simulink model "DiagnosPipelineLogical"  (R2023b)
settings: Solver=VariableStepAuto  StartTime=0.0  StopTime=10.0  RelTol=1e-3
settings Model: Creator=user  LastModifiedBy=user

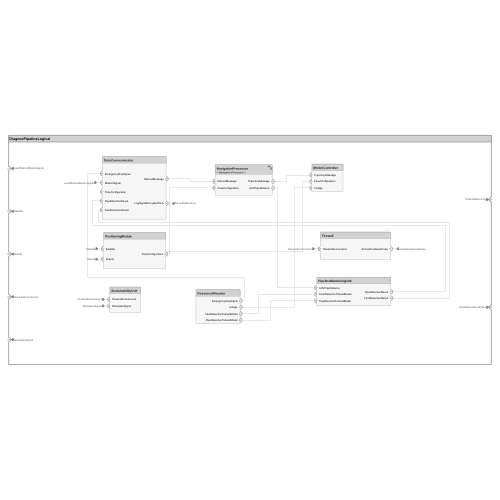
[thumbnail: Simulink's stored preview of the top-level diagram]
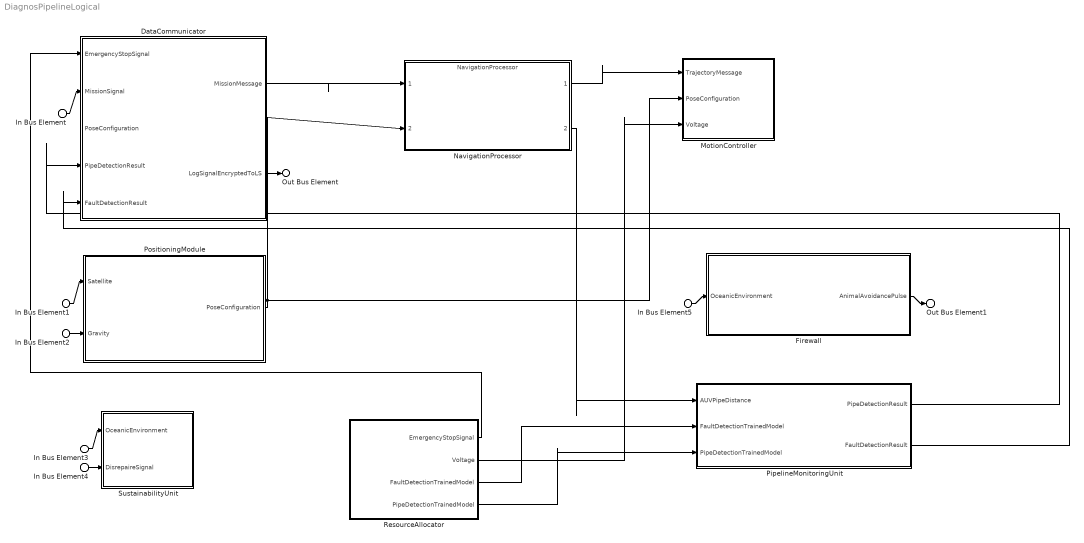
== system DiagnosPipelineLogical ==
  In Bus Element : Inport  PortName=LandStationMissionSignal
  In Bus Element1 : Inport  Port=2  PortName=Satellite
  In Bus Element2 : Inport  Port=3  PortName=Gravity
  In Bus Element3 : Inport  Port=4  PortName=OceanicEnvironment
  In Bus Element5 : Inport  Port=4  PortName=OceanicEnvironment
  In Bus Element4 : Inport  Port=5  PortName=DisrepaireSignal
  DataCommunicator : Subsystem
      settings: PortSchema="{\"entries\":[{\"content\":{\"headerSize\":26,\"margin\":15,\"minimumSpacing\":25,\"sides\":[{\"content\":{\"connectorIds\":[\"In1\",\"In2\",\"In3\",\"In4\",\"In5\"]},\"type\":\"ConnectorPlacement.EquallySpacedRectSide\",\"uuid\":\"f9fadc38-a5ed-4d2c-8740-325682f7523a\"},{\"content\":{\"connectorIds\":[\"Out1\",\"Out2\"],\"side\":\"RIGHT\"},\"type\":\"ConnectorPlacement.EquallySpacedRectSide\",\"uuid\":\"4cbd6435-b8f9-40e4-9703-696d88d9d9ae\"},{\"content\":{\"side\":\"TOP\"},\"type\":\"ConnectorPlacement.EquallySpacedRectSide\",\"uuid\":\"4cdd59a8-5a6d-4988-b682-29bfa74ce39c\"}]},\"type\":\"ConnectorPlacement.EquallySpacedConnector\",\"uuid\":\"f6db6523-916a-4ed8-a308-4b7cb9d0bc19\"}],\"packageUris\":[\"http://schema.mathworks.com/mf0/Connector/R2020b\"],\"version\":\"1.0\"}"
  Firewall : Subsystem
      settings: PortSchema="{\"entries\":[{\"content\":{\"headerSize\":26,\"margin\":15,\"minimumSpacing\":25,\"sides\":[{\"content\":{\"connectorIds\":[\"In1\"]},\"type\":\"ConnectorPlacement.EquallySpacedRectSide\",\"uuid\":\"f9fadc38-a5ed-4d2c-8740-325682f7523a\"},{\"content\":{\"connectorIds\":[\"Out1\"],\"side\":\"RIGHT\"},\"type\":\"ConnectorPlacement.EquallySpacedRectSide\",\"uuid\":\"4cbd6435-b8f9-40e4-9703-696d88d9d9ae\"},{\"content\":{\"side\":\"TOP\"},\"type\":\"ConnectorPlacement.EquallySpacedRectSide\",\"uuid\":\"4cdd59a8-5a6d-4988-b682-29bfa74ce39c\"}]},\"type\":\"ConnectorPlacement.EquallySpacedConnector\",\"uuid\":\"f6db6523-916a-4ed8-a308-4b7cb9d0bc19\"}],\"packageUris\":[\"http://schema.mathworks.com/mf0/Connector/R2020b\"],\"version\":\"1.0\"}"
  MotionController : Subsystem
      settings: PortSchema="{\"entries\":[{\"content\":{\"headerSize\":26,\"margin\":15,\"minimumSpacing\":25,\"sides\":[{\"content\":{\"connectorIds\":[\"In1\",\"In2\",\"In3\"]},\"type\":\"ConnectorPlacement.EquallySpacedRectSide\",\"uuid\":\"f9fadc38-a5ed-4d2c-8740-325682f7523a\"},{\"content\":{\"side\":\"RIGHT\"},\"type\":\"ConnectorPlacement.EquallySpacedRectSide\",\"uuid\":\"4cbd6435-b8f9-40e4-9703-696d88d9d9ae\"},{\"content\":{\"side\":\"TOP\"},\"type\":\"ConnectorPlacement.EquallySpacedRectSide\",\"uuid\":\"4cdd59a8-5a6d-4988-b682-29bfa74ce39c\"}]},\"type\":\"ConnectorPlacement.EquallySpacedConnector\",\"uuid\":\"f6db6523-916a-4ed8-a308-4b7cb9d0bc19\"}],\"packageUris\":[\"http://schema.mathworks.com/mf0/Connector/R2020b\"],\"version\":\"1.0\"}"
  NavigationProcessor : ModelReference  ModelNameDialog=NavigationProcessor  SimulationMode=Normal  ModelReferenceVersion=1.6
      settings: PortSchema="{\"entries\":[{\"content\":{\"headerSize\":38,\"margin\":15,\"minimumSpacing\":25,\"sides\":[{\"content\":{\"connectorIds\":[\"In1\",\"In2\"]},\"type\":\"ConnectorPlacement.EquallySpacedRectSide\",\"uuid\":\"f9fadc38-a5ed-4d2c-8740-325682f7523a\"},{\"content\":{\"connectorIds\":[\"Out1\",\"Out2\"],\"side\":\"RIGHT\"},\"type\":\"ConnectorPlacement.EquallySpacedRectSide\",\"uuid\":\"4cbd6435-b8f9-40e4-9703-696d88d9d9ae\"},{\"content\":{\"side\":\"TOP\"},\"type\":\"ConnectorPlacement.EquallySpacedRectSide\",\"uuid\":\"4cdd59a8-5a6d-4988-b682-29bfa74ce39c\"}]},\"type\":\"ConnectorPlacement.EquallySpacedConnector\",\"uuid\":\"f6db6523-916a-4ed8-a308-4b7cb9d0bc19\"}],\"packageUris\":[\"http://schema.mathworks.com/mf0/Connector/R2020b\"],\"version\":\"1.0\"}"
  PipelineMonitoringUnit : Subsystem
      settings: PortSchema="{\"entries\":[{\"content\":{\"headerSize\":26,\"margin\":15,\"minimumSpacing\":25,\"sides\":[{\"content\":{\"connectorIds\":[\"In1\",\"In2\",\"In3\"]},\"type\":\"ConnectorPlacement.EquallySpacedRectSide\",\"uuid\":\"f9fadc38-a5ed-4d2c-8740-325682f7523a\"},{\"content\":{\"connectorIds\":[\"Out1\",\"Out2\"],\"side\":\"RIGHT\"},\"type\":\"ConnectorPlacement.EquallySpacedRectSide\",\"uuid\":\"4cbd6435-b8f9-40e4-9703-696d88d9d9ae\"},{\"content\":{\"side\":\"TOP\"},\"type\":\"ConnectorPlacement.EquallySpacedRectSide\",\"uuid\":\"4cdd59a8-5a6d-4988-b682-29bfa74ce39c\"}]},\"type\":\"ConnectorPlacement.EquallySpacedConnector\",\"uuid\":\"f6db6523-916a-4ed8-a308-4b7cb9d0bc19\"}],\"packageUris\":[\"http://schema.mathworks.com/mf0/Connector/R2020b\"],\"version\":\"1.0\"}"
  PositioningModule : Subsystem
      settings: PortSchema="{\"entries\":[{\"content\":{\"headerSize\":26,\"margin\":15,\"minimumSpacing\":25,\"sides\":[{\"content\":{\"connectorIds\":[\"In1\",\"In2\"]},\"type\":\"ConnectorPlacement.EquallySpacedRectSide\",\"uuid\":\"f9fadc38-a5ed-4d2c-8740-325682f7523a\"},{\"content\":{\"connectorIds\":[\"Out1\"],\"side\":\"RIGHT\"},\"type\":\"ConnectorPlacement.EquallySpacedRectSide\",\"uuid\":\"4cbd6435-b8f9-40e4-9703-696d88d9d9ae\"},{\"content\":{\"side\":\"TOP\"},\"type\":\"ConnectorPlacement.EquallySpacedRectSide\",\"uuid\":\"4cdd59a8-5a6d-4988-b682-29bfa74ce39c\"}]},\"type\":\"ConnectorPlacement.EquallySpacedConnector\",\"uuid\":\"f6db6523-916a-4ed8-a308-4b7cb9d0bc19\"}],\"packageUris\":[\"http://schema.mathworks.com/mf0/Connector/R2020b\"],\"version\":\"1.0\"}"
  ResourceAllocator : Subsystem
      settings: PortSchema="{\"entries\":[{\"content\":{\"headerSize\":26,\"margin\":15,\"minimumSpacing\":25,\"sides\":[{\"content\":{},\"type\":\"ConnectorPlacement.EquallySpacedRectSide\",\"uuid\":\"f9fadc38-a5ed-4d2c-8740-325682f7523a\"},{\"content\":{\"connectorIds\":[\"Out3\",\"Out2\",\"Out1\",\"Out4\"],\"side\":\"RIGHT\"},\"type\":\"ConnectorPlacement.EquallySpacedRectSide\",\"uuid\":\"4cbd6435-b8f9-40e4-9703-696d88d9d9ae\"},{\"content\":{\"side\":\"TOP\"},\"type\":\"ConnectorPlacement.EquallySpacedRectSide\",\"uuid\":\"4cdd59a8-5a6d-4988-b682-29bfa74ce39c\"}]},\"type\":\"ConnectorPlacement.EquallySpacedConnector\",\"uuid\":\"f6db6523-916a-4ed8-a308-4b7cb9d0bc19\"}],\"packageUris\":[\"http://schema.mathworks.com/mf0/Connector/R2020b\"],\"version\":\"1.0\"}"
  SustainabilityUnit : Subsystem
      settings: PortSchema="{\"entries\":[{\"content\":{\"headerSize\":26,\"margin\":15,\"minimumSpacing\":25,\"sides\":[{\"content\":{\"connectorIds\":[\"In1\",\"In2\"]},\"type\":\"ConnectorPlacement.EquallySpacedRectSide\",\"uuid\":\"f9fadc38-a5ed-4d2c-8740-325682f7523a\"},{\"content\":{\"side\":\"RIGHT\"},\"type\":\"ConnectorPlacement.EquallySpacedRectSide\",\"uuid\":\"4cbd6435-b8f9-40e4-9703-696d88d9d9ae\"},{\"content\":{\"side\":\"TOP\"},\"type\":\"ConnectorPlacement.EquallySpacedRectSide\",\"uuid\":\"4cdd59a8-5a6d-4988-b682-29bfa74ce39c\"}]},\"type\":\"ConnectorPlacement.EquallySpacedConnector\",\"uuid\":\"f6db6523-916a-4ed8-a308-4b7cb9d0bc19\"}],\"packageUris\":[\"http://schema.mathworks.com/mf0/Connector/R2020b\"],\"version\":\"1.0\"}"
  Out Bus Element : Outport  PortName=ToLandStationLog
  Out Bus Element1 : Outport  Port=2  PortName=AnimalAvoidancePulse
  wires:
  In Bus Element/1 -> DataCommunicator/2(MissionSignal)
  DataCommunicator/2(LogSignalEncryptedToLS) -> Out Bus Element/1
  In Bus Element1/1 -> PositioningModule/1(Satellite)
  In Bus Element2/1 -> PositioningModule/2(Gravity)
  PositioningModule/1(PoseConfiguration) -> MotionController/2(PoseConfiguration), NavigationProcessor/2
  In Bus Element3/1 -> SustainabilityUnit/1(OceanicEnvironment)
  In Bus Element4/1 -> SustainabilityUnit/2(DisrepaireSignal)
  ResourceAllocator/2(Voltage) -> MotionController/3(Voltage)
  ResourceAllocator/3(EmergencyStopSignal) -> DataCommunicator/1(EmergencyStopSignal)
  ResourceAllocator/1(FaultDetectionTrainedModel) -> PipelineMonitoringUnit/2(FaultDetectionTrainedModel)
  ResourceAllocator/4(PipeDetectionTrainedModel) -> PipelineMonitoringUnit/3(PipeDetectionTrainedModel)
  PipelineMonitoringUnit/1(PipeDetectionResult) -> DataCommunicator/4(PipeDetectionResult)
  PipelineMonitoringUnit/2(FaultDetectionResult) -> DataCommunicator/5(FaultDetectionResult)
  In Bus Element5/1 -> Firewall/1(OceanicEnvironment)
  Firewall/1(AnimalAvoidancePulse) -> Out Bus Element1/1
  DataCommunicator/1(MissionMessage) -> NavigationProcessor/1
  NavigationProcessor/2 -> PipelineMonitoringUnit/1(AUVPipeDistance)
  NavigationProcessor/1 -> MotionController/1(TrajectoryMessage)

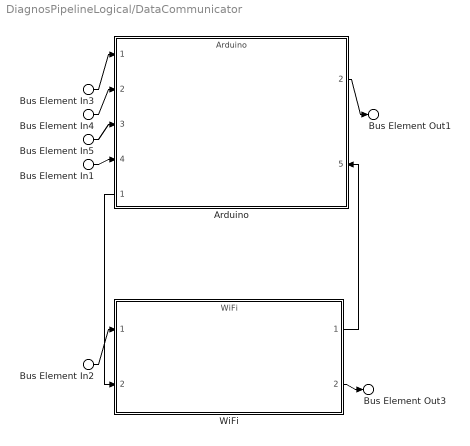
== system DiagnosPipelineLogical/DataCommunicator ==
  Bus Element In1 : Inport  PortName=EmergencyStopSignal
  Bus Element In2 : Inport  Port=2  PortName=MissionSignal
  Bus Element In3 : Inport  Port=3  PortName=PoseConfiguration
  Bus Element In4 : Inport  Port=4  PortName=PipeDetectionResult
  Bus Element In5 : Inport  Port=5  PortName=FaultDetectionResult
  Arduino : ModelReference  ModelNameDialog=Arduino  SimulationMode=Normal  ModelReferenceVersion=1.17
      settings: PortSchema="{\"entries\":[{\"content\":{\"headerSize\":38,\"margin\":15,\"minimumSpacing\":25,\"sides\":[{\"content\":{\"connectorIds\":[\"In1\",\"In2\",\"In3\",\"In4\",\"Out1\"]},\"type\":\"ConnectorPlacement.EquallySpacedRectSide\",\"uuid\":\"f9fadc38-a5ed-4d2c-8740-325682f7523a\"},{\"content\":{\"connectorIds\":[\"Out2\",\"In5\"],\"side\":\"RIGHT\"},\"type\":\"ConnectorPlacement.EquallySpacedRectSide\",\"uuid\":\"4cbd6435-b8f9-40e4-9703-696d88d9d9ae\"},{\"content\":{\"side\":\"TOP\"},\"type\":\"ConnectorPlacement.EquallySpacedRectSide\",\"uuid\":\"4cdd59a8-5a6d-4988-b682-29bfa74ce39c\"}]},\"type\":\"ConnectorPlacement.EquallySpacedConnector\",\"uuid\":\"f6db6523-916a-4ed8-a308-4b7cb9d0bc19\"}],\"packageUris\":[\"http://schema.mathworks.com/mf0/Connector/R2020b\"],\"version\":\"1.0\"}"
  WiFi : ModelReference  ModelNameDialog=WiFi  SimulationMode=Normal  ModelReferenceVersion=1.2
      settings: PortSchema="{\"entries\":[{\"content\":{\"headerSize\":38,\"margin\":15,\"minimumSpacing\":25,\"sides\":[{\"content\":{\"connectorIds\":[\"In1\",\"In2\"]},\"type\":\"ConnectorPlacement.EquallySpacedRectSide\",\"uuid\":\"f9fadc38-a5ed-4d2c-8740-325682f7523a\"},{\"content\":{\"connectorIds\":[\"Out1\",\"Out2\"],\"side\":\"RIGHT\"},\"type\":\"ConnectorPlacement.EquallySpacedRectSide\",\"uuid\":\"4cbd6435-b8f9-40e4-9703-696d88d9d9ae\"},{\"content\":{\"side\":\"TOP\"},\"type\":\"ConnectorPlacement.EquallySpacedRectSide\",\"uuid\":\"4cdd59a8-5a6d-4988-b682-29bfa74ce39c\"}]},\"type\":\"ConnectorPlacement.EquallySpacedConnector\",\"uuid\":\"f6db6523-916a-4ed8-a308-4b7cb9d0bc19\"}],\"packageUris\":[\"http://schema.mathworks.com/mf0/Connector/R2020b\"],\"version\":\"1.0\"}"
  Bus Element Out1 : Outport  PortName=MissionMessage
  Bus Element Out3 : Outport  Port=2  PortName=LogSignalEncryptedToLS
  wires:
  Bus Element In1/1 -> Arduino/4
  Bus Element In5/1 -> Arduino/3
  Bus Element In4/1 -> Arduino/2
  Bus Element In3/1 -> Arduino/1
  Arduino/2 -> Bus Element Out1/1
  Arduino/1 -> WiFi/2
  Bus Element In2/1 -> WiFi/1
  WiFi/2 -> Bus Element Out3/1
  WiFi/1 -> Arduino/5

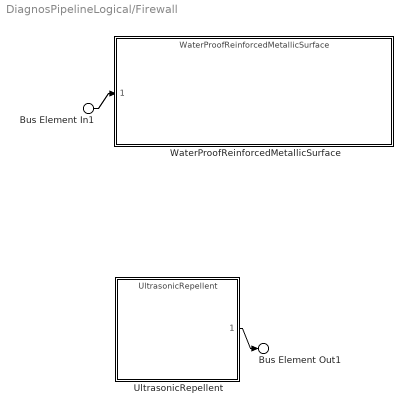
== system DiagnosPipelineLogical/Firewall ==
  Bus Element In1 : Inport  PortName=OceanicEnvironment
  UltrasonicRepellent : ModelReference  ModelNameDialog=UltrasonicRepellent  SimulationMode=Normal  ModelReferenceVersion=1.2
      settings: PortSchema="{\"entries\":[{\"content\":{\"headerSize\":38,\"margin\":15,\"minimumSpacing\":25,\"sides\":[{\"content\":{},\"type\":\"ConnectorPlacement.EquallySpacedRectSide\",\"uuid\":\"f9fadc38-a5ed-4d2c-8740-325682f7523a\"},{\"content\":{\"connectorIds\":[\"Out1\"],\"side\":\"RIGHT\"},\"type\":\"ConnectorPlacement.EquallySpacedRectSide\",\"uuid\":\"4cbd6435-b8f9-40e4-9703-696d88d9d9ae\"},{\"content\":{\"side\":\"TOP\"},\"type\":\"ConnectorPlacement.EquallySpacedRectSide\",\"uuid\":\"4cdd59a8-5a6d-4988-b682-29bfa74ce39c\"}]},\"type\":\"ConnectorPlacement.EquallySpacedConnector\",\"uuid\":\"f6db6523-916a-4ed8-a308-4b7cb9d0bc19\"}],\"packageUris\":[\"http://schema.mathworks.com/mf0/Connector/R2020b\"],\"version\":\"1.0\"}"
  WaterProofReinforcedMetallicSurface : ModelReference  ModelNameDialog=WaterProofReinforcedMetallicSurface  SimulationMode=Normal  ModelReferenceVersion=1.1
      settings: PortSchema="{\"entries\":[{\"content\":{\"headerSize\":38,\"margin\":15,\"minimumSpacing\":25,\"sides\":[{\"content\":{\"connectorIds\":[\"In1\"]},\"type\":\"ConnectorPlacement.EquallySpacedRectSide\",\"uuid\":\"f9fadc38-a5ed-4d2c-8740-325682f7523a\"},{\"content\":{\"side\":\"RIGHT\"},\"type\":\"ConnectorPlacement.EquallySpacedRectSide\",\"uuid\":\"4cbd6435-b8f9-40e4-9703-696d88d9d9ae\"},{\"content\":{\"side\":\"TOP\"},\"type\":\"ConnectorPlacement.EquallySpacedRectSide\",\"uuid\":\"4cdd59a8-5a6d-4988-b682-29bfa74ce39c\"}]},\"type\":\"ConnectorPlacement.EquallySpacedConnector\",\"uuid\":\"f6db6523-916a-4ed8-a308-4b7cb9d0bc19\"}],\"packageUris\":[\"http://schema.mathworks.com/mf0/Connector/R2020b\"],\"version\":\"1.0\"}"
  Bus Element Out1 : Outport  PortName=AnimalAvoidancePulse
  wires:
  Bus Element In1/1 -> WaterProofReinforcedMetallicSurface/1
  UltrasonicRepellent/1 -> Bus Element Out1/1

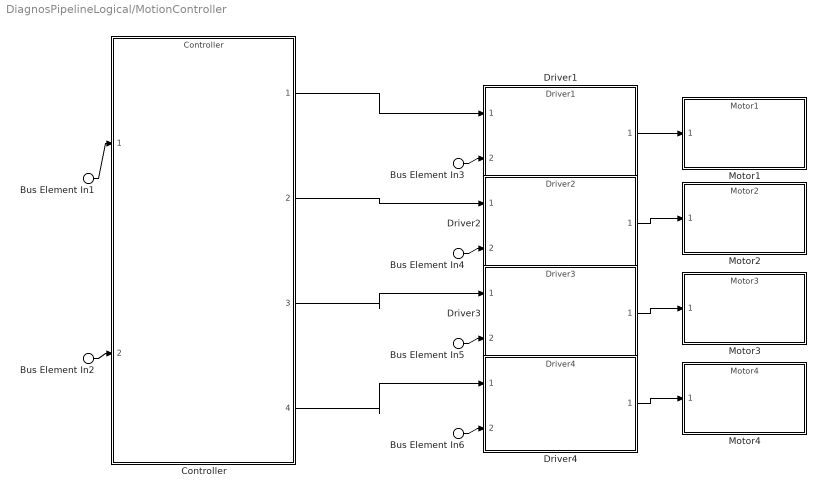
== system DiagnosPipelineLogical/MotionController ==
  Bus Element In1 : Inport  PortName=TrajectoryMessage
  Bus Element In2 : Inport  Port=2  PortName=PoseConfiguration
  Bus Element In{3..6} (4 alike) : Inport  Port=3  PortName=Voltage
  Controller : ModelReference  ModelNameDialog=Controller  SimulationMode=Normal  ModelReferenceVersion=1.2
      settings: PortSchema="{\"entries\":[{\"content\":{\"headerSize\":38,\"margin\":15,\"minimumSpacing\":25,\"sides\":[{\"content\":{\"connectorIds\":[\"In1\",\"In2\"]},\"type\":\"ConnectorPlacement.EquallySpacedRectSide\",\"uuid\":\"f9fadc38-a5ed-4d2c-8740-325682f7523a\"},{\"content\":{\"connectorIds\":[\"Out1\",\"Out2\",\"Out3\",\"Out4\"],\"side\":\"RIGHT\"},\"type\":\"ConnectorPlacement.EquallySpacedRectSide\",\"uuid\":\"4cbd6435-b8f9-40e4-9703-696d88d9d9ae\"},{\"content\":{\"side\":\"TOP\"},\"type\":\"ConnectorPlacement.EquallySpacedRectSide\",\"uuid\":\"4cdd59a8-5a6d-4988-b682-29bfa74ce39c\"}]},\"type\":\"ConnectorPlacement.EquallySpacedConnector\",\"uuid\":\"f6db6523-916a-4ed8-a308-4b7cb9d0bc19\"}],\"packageUris\":[\"http://schema.mathworks.com/mf0/Connector/R2020b\"],\"version\":\"1.0\"}"
  Driver1 : ModelReference  ModelNameDialog=Driver1  SimulationMode=Normal  ModelReferenceVersion=1.2
      settings: PortSchema="{\"entries\":[{\"content\":{\"headerSize\":38,\"margin\":15,\"minimumSpacing\":25,\"sides\":[{\"content\":{\"connectorIds\":[\"In1\",\"In2\"]},\"type\":\"ConnectorPlacement.EquallySpacedRectSide\",\"uuid\":\"f9fadc38-a5ed-4d2c-8740-325682f7523a\"},{\"content\":{\"connectorIds\":[\"Out1\"],\"side\":\"RIGHT\"},\"type\":\"ConnectorPlacement.EquallySpacedRectSide\",\"uuid\":\"4cbd6435-b8f9-40e4-9703-696d88d9d9ae\"},{\"content\":{\"side\":\"TOP\"},\"type\":\"ConnectorPlacement.EquallySpacedRectSide\",\"uuid\":\"4cdd59a8-5a6d-4988-b682-29bfa74ce39c\"}]},\"type\":\"ConnectorPlacement.EquallySpacedConnector\",\"uuid\":\"f6db6523-916a-4ed8-a308-4b7cb9d0bc19\"}],\"packageUris\":[\"http://schema.mathworks.com/mf0/Connector/R2020b\"],\"version\":\"1.0\"}"
  Driver2 : ModelReference  ModelNameDialog=Driver2  SimulationMode=Normal  ModelReferenceVersion=1.2
      settings: PortSchema="{\"entries\":[{\"content\":{\"headerSize\":38,\"margin\":15,\"minimumSpacing\":25,\"sides\":[{\"content\":{\"connectorIds\":[\"In1\",\"In2\"]},\"type\":\"ConnectorPlacement.EquallySpacedRectSide\",\"uuid\":\"f9fadc38-a5ed-4d2c-8740-325682f7523a\"},{\"content\":{\"connectorIds\":[\"Out1\"],\"side\":\"RIGHT\"},\"type\":\"ConnectorPlacement.EquallySpacedRectSide\",\"uuid\":\"4cbd6435-b8f9-40e4-9703-696d88d9d9ae\"},{\"content\":{\"side\":\"TOP\"},\"type\":\"ConnectorPlacement.EquallySpacedRectSide\",\"uuid\":\"4cdd59a8-5a6d-4988-b682-29bfa74ce39c\"}]},\"type\":\"ConnectorPlacement.EquallySpacedConnector\",\"uuid\":\"f6db6523-916a-4ed8-a308-4b7cb9d0bc19\"}],\"packageUris\":[\"http://schema.mathworks.com/mf0/Connector/R2020b\"],\"version\":\"1.0\"}"
  Driver3 : ModelReference  ModelNameDialog=Driver3  SimulationMode=Normal  ModelReferenceVersion=1.3
      settings: PortSchema="{\"entries\":[{\"content\":{\"headerSize\":38,\"margin\":15,\"minimumSpacing\":25,\"sides\":[{\"content\":{\"connectorIds\":[\"In1\",\"In2\"]},\"type\":\"ConnectorPlacement.EquallySpacedRectSide\",\"uuid\":\"f9fadc38-a5ed-4d2c-8740-325682f7523a\"},{\"content\":{\"connectorIds\":[\"Out1\"],\"side\":\"RIGHT\"},\"type\":\"ConnectorPlacement.EquallySpacedRectSide\",\"uuid\":\"4cbd6435-b8f9-40e4-9703-696d88d9d9ae\"},{\"content\":{\"side\":\"TOP\"},\"type\":\"ConnectorPlacement.EquallySpacedRectSide\",\"uuid\":\"4cdd59a8-5a6d-4988-b682-29bfa74ce39c\"}]},\"type\":\"ConnectorPlacement.EquallySpacedConnector\",\"uuid\":\"f6db6523-916a-4ed8-a308-4b7cb9d0bc19\"}],\"packageUris\":[\"http://schema.mathworks.com/mf0/Connector/R2020b\"],\"version\":\"1.0\"}"
  Driver4 : ModelReference  ModelNameDialog=Driver4  SimulationMode=Normal  ModelReferenceVersion=1.2
      settings: PortSchema="{\"entries\":[{\"content\":{\"headerSize\":38,\"margin\":15,\"minimumSpacing\":25,\"sides\":[{\"content\":{\"connectorIds\":[\"In1\",\"In2\"]},\"type\":\"ConnectorPlacement.EquallySpacedRectSide\",\"uuid\":\"f9fadc38-a5ed-4d2c-8740-325682f7523a\"},{\"content\":{\"connectorIds\":[\"Out1\"],\"side\":\"RIGHT\"},\"type\":\"ConnectorPlacement.EquallySpacedRectSide\",\"uuid\":\"4cbd6435-b8f9-40e4-9703-696d88d9d9ae\"},{\"content\":{\"side\":\"TOP\"},\"type\":\"ConnectorPlacement.EquallySpacedRectSide\",\"uuid\":\"4cdd59a8-5a6d-4988-b682-29bfa74ce39c\"}]},\"type\":\"ConnectorPlacement.EquallySpacedConnector\",\"uuid\":\"f6db6523-916a-4ed8-a308-4b7cb9d0bc19\"}],\"packageUris\":[\"http://schema.mathworks.com/mf0/Connector/R2020b\"],\"version\":\"1.0\"}"
  Motor1 : ModelReference  ModelNameDialog=Motor1  SimulationMode=Normal  ModelReferenceVersion=1.2
      settings: PortSchema="{\"entries\":[{\"content\":{\"headerSize\":38,\"margin\":15,\"minimumSpacing\":25,\"sides\":[{\"content\":{\"connectorIds\":[\"In1\"]},\"type\":\"ConnectorPlacement.EquallySpacedRectSide\",\"uuid\":\"f9fadc38-a5ed-4d2c-8740-325682f7523a\"},{\"content\":{\"side\":\"RIGHT\"},\"type\":\"ConnectorPlacement.EquallySpacedRectSide\",\"uuid\":\"4cbd6435-b8f9-40e4-9703-696d88d9d9ae\"},{\"content\":{\"side\":\"TOP\"},\"type\":\"ConnectorPlacement.EquallySpacedRectSide\",\"uuid\":\"4cdd59a8-5a6d-4988-b682-29bfa74ce39c\"}]},\"type\":\"ConnectorPlacement.EquallySpacedConnector\",\"uuid\":\"f6db6523-916a-4ed8-a308-4b7cb9d0bc19\"}],\"packageUris\":[\"http://schema.mathworks.com/mf0/Connector/R2020b\"],\"version\":\"1.0\"}"
  Motor2 : ModelReference  ModelNameDialog=Motor2  SimulationMode=Normal  ModelReferenceVersion=1.2
      settings: PortSchema="{\"entries\":[{\"content\":{\"headerSize\":38,\"margin\":15,\"minimumSpacing\":25,\"sides\":[{\"content\":{\"connectorIds\":[\"In1\"]},\"type\":\"ConnectorPlacement.EquallySpacedRectSide\",\"uuid\":\"f9fadc38-a5ed-4d2c-8740-325682f7523a\"},{\"content\":{\"side\":\"RIGHT\"},\"type\":\"ConnectorPlacement.EquallySpacedRectSide\",\"uuid\":\"4cbd6435-b8f9-40e4-9703-696d88d9d9ae\"},{\"content\":{\"side\":\"TOP\"},\"type\":\"ConnectorPlacement.EquallySpacedRectSide\",\"uuid\":\"4cdd59a8-5a6d-4988-b682-29bfa74ce39c\"}]},\"type\":\"ConnectorPlacement.EquallySpacedConnector\",\"uuid\":\"f6db6523-916a-4ed8-a308-4b7cb9d0bc19\"}],\"packageUris\":[\"http://schema.mathworks.com/mf0/Connector/R2020b\"],\"version\":\"1.0\"}"
  Motor3 : ModelReference  ModelNameDialog=Motor3  SimulationMode=Normal  ModelReferenceVersion=1.2
      settings: PortSchema="{\"entries\":[{\"content\":{\"headerSize\":38,\"margin\":15,\"minimumSpacing\":25,\"sides\":[{\"content\":{\"connectorIds\":[\"In1\"]},\"type\":\"ConnectorPlacement.EquallySpacedRectSide\",\"uuid\":\"f9fadc38-a5ed-4d2c-8740-325682f7523a\"},{\"content\":{\"side\":\"RIGHT\"},\"type\":\"ConnectorPlacement.EquallySpacedRectSide\",\"uuid\":\"4cbd6435-b8f9-40e4-9703-696d88d9d9ae\"},{\"content\":{\"side\":\"TOP\"},\"type\":\"ConnectorPlacement.EquallySpacedRectSide\",\"uuid\":\"4cdd59a8-5a6d-4988-b682-29bfa74ce39c\"}]},\"type\":\"ConnectorPlacement.EquallySpacedConnector\",\"uuid\":\"f6db6523-916a-4ed8-a308-4b7cb9d0bc19\"}],\"packageUris\":[\"http://schema.mathworks.com/mf0/Connector/R2020b\"],\"version\":\"1.0\"}"
  Motor4 : ModelReference  ModelNameDialog=Motor4  SimulationMode=Normal  ModelReferenceVersion=1.2
      settings: PortSchema="{\"entries\":[{\"content\":{\"headerSize\":38,\"margin\":15,\"minimumSpacing\":25,\"sides\":[{\"content\":{\"connectorIds\":[\"In1\"]},\"type\":\"ConnectorPlacement.EquallySpacedRectSide\",\"uuid\":\"f9fadc38-a5ed-4d2c-8740-325682f7523a\"},{\"content\":{\"side\":\"RIGHT\"},\"type\":\"ConnectorPlacement.EquallySpacedRectSide\",\"uuid\":\"4cbd6435-b8f9-40e4-9703-696d88d9d9ae\"},{\"content\":{\"side\":\"TOP\"},\"type\":\"ConnectorPlacement.EquallySpacedRectSide\",\"uuid\":\"4cdd59a8-5a6d-4988-b682-29bfa74ce39c\"}]},\"type\":\"ConnectorPlacement.EquallySpacedConnector\",\"uuid\":\"f6db6523-916a-4ed8-a308-4b7cb9d0bc19\"}],\"packageUris\":[\"http://schema.mathworks.com/mf0/Connector/R2020b\"],\"version\":\"1.0\"}"
  wires:
  Bus Element In2/1 -> Controller/2
  Bus Element In1/1 -> Controller/1
  Controller/1 -> Driver1/1
  Bus Element In3/1 -> Driver1/2
  Controller/2 -> Driver2/1
  Bus Element In4/1 -> Driver2/2
  Controller/3 -> Driver3/1
  Bus Element In5/1 -> Driver3/2
  Controller/4 -> Driver4/1
  Bus Element In6/1 -> Driver4/2
  Driver1/1 -> Motor1/1
  Driver2/1 -> Motor2/1
  Driver3/1 -> Motor3/1
  Driver4/1 -> Motor4/1

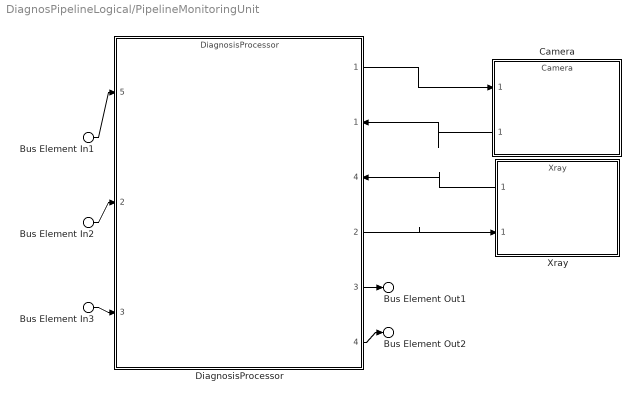
== system DiagnosPipelineLogical/PipelineMonitoringUnit ==
  Bus Element In1 : Inport  PortName=AUVPipeDistance
  Bus Element In2 : Inport  Port=2  PortName=FaultDetectionTrainedModel
  Bus Element In3 : Inport  Port=3  PortName=PipeDetectionTrainedModel
  Camera : ModelReference  ModelNameDialog=Camera  SimulationMode=Normal  ModelReferenceVersion=1.4
      settings: PortSchema="{\"entries\":[{\"content\":{\"headerSize\":38,\"margin\":15,\"minimumSpacing\":25,\"sides\":[{\"content\":{\"connectorIds\":[\"In1\",\"Out1\"]},\"type\":\"ConnectorPlacement.EquallySpacedRectSide\",\"uuid\":\"f9fadc38-a5ed-4d2c-8740-325682f7523a\"},{\"content\":{\"side\":\"RIGHT\"},\"type\":\"ConnectorPlacement.EquallySpacedRectSide\",\"uuid\":\"4cbd6435-b8f9-40e4-9703-696d88d9d9ae\"},{\"content\":{\"side\":\"TOP\"},\"type\":\"ConnectorPlacement.EquallySpacedRectSide\",\"uuid\":\"4cdd59a8-5a6d-4988-b682-29bfa74ce39c\"}]},\"type\":\"ConnectorPlacement.EquallySpacedConnector\",\"uuid\":\"f6db6523-916a-4ed8-a308-4b7cb9d0bc19\"}],\"packageUris\":[\"http://schema.mathworks.com/mf0/Connector/R2020b\"],\"version\":\"1.0\"}"
  DiagnosisProcessor : ModelReference  ModelNameDialog=DiagnosisProcessor  SimulationMode=Normal  ModelReferenceVersion=1.3
      settings: PortSchema="{\"entries\":[{\"content\":{\"headerSize\":38,\"margin\":15,\"minimumSpacing\":25,\"sides\":[{\"content\":{\"connectorIds\":[\"In5\",\"In2\",\"In3\"]},\"type\":\"ConnectorPlacement.EquallySpacedRectSide\",\"uuid\":\"f9fadc38-a5ed-4d2c-8740-325682f7523a\"},{\"content\":{\"connectorIds\":[\"Out1\",\"In1\",\"In4\",\"Out2\",\"Out3\",\"Out4\"],\"side\":\"RIGHT\"},\"type\":\"ConnectorPlacement.EquallySpacedRectSide\",\"uuid\":\"4cbd6435-b8f9-40e4-9703-696d88d9d9ae\"},{\"content\":{\"side\":\"TOP\"},\"type\":\"ConnectorPlacement.EquallySpacedRectSide\",\"uuid\":\"4cdd59a8-5a6d-4988-b682-29bfa74ce39c\"}]},\"type\":\"ConnectorPlacement.EquallySpacedConnector\",\"uuid\":\"f6db6523-916a-4ed8-a308-4b7cb9d0bc19\"}],\"packageUris\":[\"http://schema.mathworks.com/mf0/Connector/R2020b\"],\"version\":\"1.0\"}"
  Xray : ModelReference  ModelNameDialog=Xray  SimulationMode=Normal  ModelReferenceVersion=1.2
      settings: PortSchema="{\"entries\":[{\"content\":{\"headerSize\":38,\"margin\":15,\"minimumSpacing\":25,\"sides\":[{\"content\":{\"connectorIds\":[\"Out1\",\"In1\"]},\"type\":\"ConnectorPlacement.EquallySpacedRectSide\",\"uuid\":\"f9fadc38-a5ed-4d2c-8740-325682f7523a\"},{\"content\":{\"side\":\"RIGHT\"},\"type\":\"ConnectorPlacement.EquallySpacedRectSide\",\"uuid\":\"4cbd6435-b8f9-40e4-9703-696d88d9d9ae\"},{\"content\":{\"side\":\"TOP\"},\"type\":\"ConnectorPlacement.EquallySpacedRectSide\",\"uuid\":\"4cdd59a8-5a6d-4988-b682-29bfa74ce39c\"}]},\"type\":\"ConnectorPlacement.EquallySpacedConnector\",\"uuid\":\"f6db6523-916a-4ed8-a308-4b7cb9d0bc19\"}],\"packageUris\":[\"http://schema.mathworks.com/mf0/Connector/R2020b\"],\"version\":\"1.0\"}"
  Bus Element Out1 : Outport  PortName=PipeDetectionResult
  Bus Element Out2 : Outport  Port=2  PortName=FaultDetectionResult
  wires:
  Bus Element In1/1 -> DiagnosisProcessor/5
  Bus Element In2/1 -> DiagnosisProcessor/2
  Bus Element In3/1 -> DiagnosisProcessor/3
  DiagnosisProcessor/4 -> Bus Element Out2/1
  DiagnosisProcessor/3 -> Bus Element Out1/1
  DiagnosisProcessor/1 -> Camera/1
  Camera/1 -> DiagnosisProcessor/1
  DiagnosisProcessor/2 -> Xray/1
  Xray/1 -> DiagnosisProcessor/4

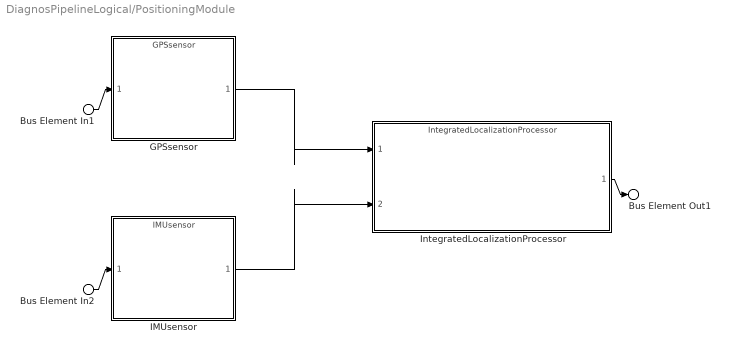
== system DiagnosPipelineLogical/PositioningModule ==
  Bus Element In1 : Inport  PortName=Satellite
  Bus Element In2 : Inport  Port=2  PortName=Gravity
  GPSsensor : ModelReference  ModelNameDialog=GPSsensor  SimulationMode=Normal  ModelReferenceVersion=1.3
      settings: PortSchema="{\"entries\":[{\"content\":{\"headerSize\":38,\"margin\":15,\"minimumSpacing\":25,\"sides\":[{\"content\":{\"connectorIds\":[\"In1\"]},\"type\":\"ConnectorPlacement.EquallySpacedRectSide\",\"uuid\":\"f9fadc38-a5ed-4d2c-8740-325682f7523a\"},{\"content\":{\"connectorIds\":[\"Out1\"],\"side\":\"RIGHT\"},\"type\":\"ConnectorPlacement.EquallySpacedRectSide\",\"uuid\":\"4cbd6435-b8f9-40e4-9703-696d88d9d9ae\"},{\"content\":{\"side\":\"TOP\"},\"type\":\"ConnectorPlacement.EquallySpacedRectSide\",\"uuid\":\"4cdd59a8-5a6d-4988-b682-29bfa74ce39c\"}]},\"type\":\"ConnectorPlacement.EquallySpacedConnector\",\"uuid\":\"f6db6523-916a-4ed8-a308-4b7cb9d0bc19\"}],\"packageUris\":[\"http://schema.mathworks.com/mf0/Connector/R2020b\"],\"version\":\"1.0\"}"
  IMUsensor : ModelReference  ModelNameDialog=IMUsensor  SimulationMode=Normal  ModelReferenceVersion=1.5
      settings: PortSchema="{\"entries\":[{\"content\":{\"headerSize\":38,\"margin\":15,\"minimumSpacing\":25,\"sides\":[{\"content\":{\"connectorIds\":[\"In1\"]},\"type\":\"ConnectorPlacement.EquallySpacedRectSide\",\"uuid\":\"f9fadc38-a5ed-4d2c-8740-325682f7523a\"},{\"content\":{\"connectorIds\":[\"Out1\"],\"side\":\"RIGHT\"},\"type\":\"ConnectorPlacement.EquallySpacedRectSide\",\"uuid\":\"4cbd6435-b8f9-40e4-9703-696d88d9d9ae\"},{\"content\":{\"side\":\"TOP\"},\"type\":\"ConnectorPlacement.EquallySpacedRectSide\",\"uuid\":\"4cdd59a8-5a6d-4988-b682-29bfa74ce39c\"}]},\"type\":\"ConnectorPlacement.EquallySpacedConnector\",\"uuid\":\"f6db6523-916a-4ed8-a308-4b7cb9d0bc19\"}],\"packageUris\":[\"http://schema.mathworks.com/mf0/Connector/R2020b\"],\"version\":\"1.0\"}"
  IntegratedLocalizationProcessor : ModelReference  ModelNameDialog=IntegratedLocalizationProcessor  SimulationMode=Normal  ModelReferenceVersion=1.25
      settings: PortSchema="{\"entries\":[{\"content\":{\"headerSize\":38,\"margin\":15,\"minimumSpacing\":25,\"sides\":[{\"content\":{\"connectorIds\":[\"In1\",\"In2\"]},\"type\":\"ConnectorPlacement.EquallySpacedRectSide\",\"uuid\":\"f9fadc38-a5ed-4d2c-8740-325682f7523a\"},{\"content\":{\"connectorIds\":[\"Out1\"],\"side\":\"RIGHT\"},\"type\":\"ConnectorPlacement.EquallySpacedRectSide\",\"uuid\":\"4cbd6435-b8f9-40e4-9703-696d88d9d9ae\"},{\"content\":{\"side\":\"TOP\"},\"type\":\"ConnectorPlacement.EquallySpacedRectSide\",\"uuid\":\"4cdd59a8-5a6d-4988-b682-29bfa74ce39c\"}]},\"type\":\"ConnectorPlacement.EquallySpacedConnector\",\"uuid\":\"f6db6523-916a-4ed8-a308-4b7cb9d0bc19\"}],\"packageUris\":[\"http://schema.mathworks.com/mf0/Connector/R2020b\"],\"version\":\"1.0\"}"
  Bus Element Out1 : Outport  PortName=PoseConfiguration
  wires:
  Bus Element In1/1 -> GPSsensor/1
  Bus Element In2/1 -> IMUsensor/1
  IMUsensor/1 -> IntegratedLocalizationProcessor/2
  GPSsensor/1 -> IntegratedLocalizationProcessor/1
  IntegratedLocalizationProcessor/1 -> Bus Element Out1/1

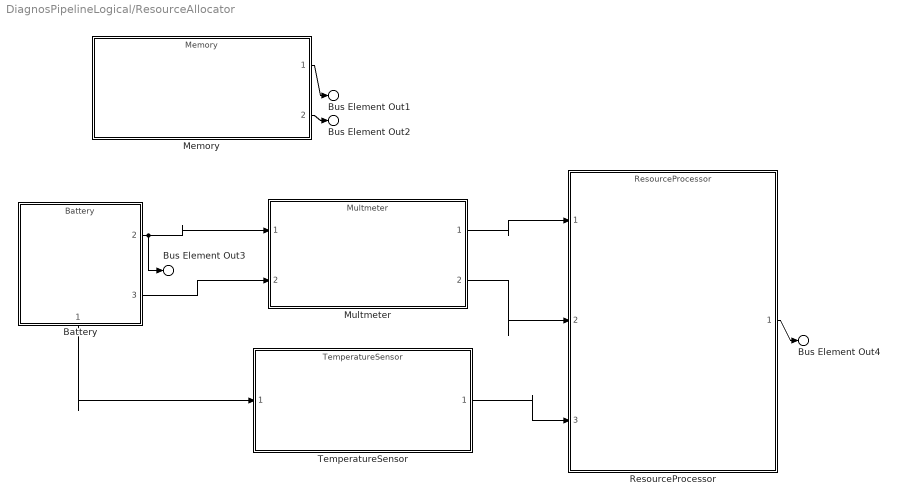
== system DiagnosPipelineLogical/ResourceAllocator ==
  Battery : ModelReference  ModelNameDialog=Battery  SimulationMode=Normal  ModelReferenceVersion=1.3
      settings: PortSchema="{\"entries\":[{\"content\":{\"headerSize\":38,\"margin\":15,\"minimumSpacing\":25,\"sides\":[{\"content\":{},\"type\":\"ConnectorPlacement.EquallySpacedRectSide\",\"uuid\":\"f9fadc38-a5ed-4d2c-8740-325682f7523a\"},{\"content\":{\"connectorIds\":[\"Out2\",\"Out3\"],\"side\":\"RIGHT\"},\"type\":\"ConnectorPlacement.EquallySpacedRectSide\",\"uuid\":\"4cbd6435-b8f9-40e4-9703-696d88d9d9ae\"},{\"content\":{\"side\":\"TOP\"},\"type\":\"ConnectorPlacement.EquallySpacedRectSide\",\"uuid\":\"4cdd59a8-5a6d-4988-b682-29bfa74ce39c\"},{\"content\":{\"connectorIds\":[\"Out1\"],\"side\":\"BOTTOM\"},\"type\":\"ConnectorPlacement.EquallySpacedRectSide\",\"uuid\":\"54b9e8e1-ed1a-443b-b89e-f595aeddcba4\"}]},\"type\":\"ConnectorPlacement.EquallySpacedConnector\",\"uuid\":\"f6db6523-916a-4ed8-a308-4b7cb9d0bc19\"}],\"packageUris\":[\"http://schema.mathworks.com/mf0/Connector/R2020b\"],\"version\":\"1.0\"}"
  Memory : ModelReference  ModelNameDialog=Memory  SimulationMode=Normal  ModelReferenceVersion=1.2
      settings: PortSchema="{\"entries\":[{\"content\":{\"headerSize\":38,\"margin\":15,\"minimumSpacing\":25,\"sides\":[{\"content\":{},\"type\":\"ConnectorPlacement.EquallySpacedRectSide\",\"uuid\":\"f9fadc38-a5ed-4d2c-8740-325682f7523a\"},{\"content\":{\"connectorIds\":[\"Out1\",\"Out2\"],\"side\":\"RIGHT\"},\"type\":\"ConnectorPlacement.EquallySpacedRectSide\",\"uuid\":\"4cbd6435-b8f9-40e4-9703-696d88d9d9ae\"},{\"content\":{\"side\":\"TOP\"},\"type\":\"ConnectorPlacement.EquallySpacedRectSide\",\"uuid\":\"4cdd59a8-5a6d-4988-b682-29bfa74ce39c\"}]},\"type\":\"ConnectorPlacement.EquallySpacedConnector\",\"uuid\":\"f6db6523-916a-4ed8-a308-4b7cb9d0bc19\"}],\"packageUris\":[\"http://schema.mathworks.com/mf0/Connector/R2020b\"],\"version\":\"1.0\"}"
  Multmeter : ModelReference  ModelNameDialog=Multmeter  SimulationMode=Normal  ModelReferenceVersion=1.2
      settings: PortSchema="{\"entries\":[{\"content\":{\"headerSize\":38,\"margin\":15,\"minimumSpacing\":25,\"sides\":[{\"content\":{\"connectorIds\":[\"In1\",\"In2\"]},\"type\":\"ConnectorPlacement.EquallySpacedRectSide\",\"uuid\":\"f9fadc38-a5ed-4d2c-8740-325682f7523a\"},{\"content\":{\"connectorIds\":[\"Out1\",\"Out2\"],\"side\":\"RIGHT\"},\"type\":\"ConnectorPlacement.EquallySpacedRectSide\",\"uuid\":\"4cbd6435-b8f9-40e4-9703-696d88d9d9ae\"},{\"content\":{\"side\":\"TOP\"},\"type\":\"ConnectorPlacement.EquallySpacedRectSide\",\"uuid\":\"4cdd59a8-5a6d-4988-b682-29bfa74ce39c\"}]},\"type\":\"ConnectorPlacement.EquallySpacedConnector\",\"uuid\":\"f6db6523-916a-4ed8-a308-4b7cb9d0bc19\"}],\"packageUris\":[\"http://schema.mathworks.com/mf0/Connector/R2020b\"],\"version\":\"1.0\"}"
  ResourceProcessor : ModelReference  ModelNameDialog=ResourceProcessor  SimulationMode=Normal  ModelReferenceVersion=1.2
      settings: PortSchema="{\"entries\":[{\"content\":{\"headerSize\":38,\"margin\":15,\"minimumSpacing\":25,\"sides\":[{\"content\":{\"connectorIds\":[\"In1\",\"In2\",\"In3\"]},\"type\":\"ConnectorPlacement.EquallySpacedRectSide\",\"uuid\":\"f9fadc38-a5ed-4d2c-8740-325682f7523a\"},{\"content\":{\"connectorIds\":[\"Out1\"],\"side\":\"RIGHT\"},\"type\":\"ConnectorPlacement.EquallySpacedRectSide\",\"uuid\":\"4cbd6435-b8f9-40e4-9703-696d88d9d9ae\"},{\"content\":{\"side\":\"TOP\"},\"type\":\"ConnectorPlacement.EquallySpacedRectSide\",\"uuid\":\"4cdd59a8-5a6d-4988-b682-29bfa74ce39c\"}]},\"type\":\"ConnectorPlacement.EquallySpacedConnector\",\"uuid\":\"f6db6523-916a-4ed8-a308-4b7cb9d0bc19\"}],\"packageUris\":[\"http://schema.mathworks.com/mf0/Connector/R2020b\"],\"version\":\"1.0\"}"
  TemperatureSensor : ModelReference  ModelNameDialog=TemperatureSensor  SimulationMode=Normal  ModelReferenceVersion=1.2
      settings: PortSchema="{\"entries\":[{\"content\":{\"headerSize\":38,\"margin\":15,\"minimumSpacing\":25,\"sides\":[{\"content\":{\"connectorIds\":[\"In1\"]},\"type\":\"ConnectorPlacement.EquallySpacedRectSide\",\"uuid\":\"f9fadc38-a5ed-4d2c-8740-325682f7523a\"},{\"content\":{\"connectorIds\":[\"Out1\"],\"side\":\"RIGHT\"},\"type\":\"ConnectorPlacement.EquallySpacedRectSide\",\"uuid\":\"4cbd6435-b8f9-40e4-9703-696d88d9d9ae\"},{\"content\":{\"side\":\"TOP\"},\"type\":\"ConnectorPlacement.EquallySpacedRectSide\",\"uuid\":\"4cdd59a8-5a6d-4988-b682-29bfa74ce39c\"}]},\"type\":\"ConnectorPlacement.EquallySpacedConnector\",\"uuid\":\"f6db6523-916a-4ed8-a308-4b7cb9d0bc19\"}],\"packageUris\":[\"http://schema.mathworks.com/mf0/Connector/R2020b\"],\"version\":\"1.0\"}"
  Bus Element Out2 : Outport  PortName=FaultDetectionTrainedModel
  Bus Element Out3 : Outport  Port=2  PortName=Voltage
  Bus Element Out4 : Outport  Port=3  PortName=EmergencyStopSignal
  Bus Element Out1 : Outport  Port=4  PortName=PipeDetectionTrainedModel
  wires:
  Memory/2 -> Bus Element Out2/1
  Memory/1 -> Bus Element Out1/1
  Battery/2 -> Bus Element Out3/1, Multmeter/1
  Battery/3 -> Multmeter/2
  Battery/1 -> TemperatureSensor/1
  Multmeter/2 -> ResourceProcessor/2
  TemperatureSensor/1 -> ResourceProcessor/3
  Multmeter/1 -> ResourceProcessor/1
  ResourceProcessor/1 -> Bus Element Out4/1

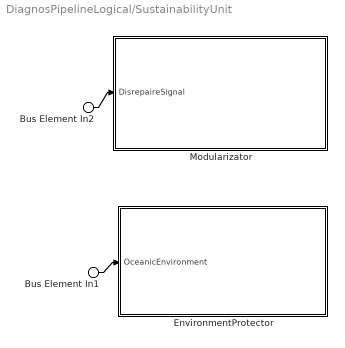
== system DiagnosPipelineLogical/SustainabilityUnit ==
  Bus Element In1 : Inport  PortName=OceanicEnvironment
  Bus Element In2 : Inport  Port=2  PortName=DisrepaireSignal
  EnvironmentProtector : Subsystem
      settings: PortSchema="{\"entries\":[{\"content\":{\"headerSize\":26,\"margin\":15,\"minimumSpacing\":25,\"sides\":[{\"content\":{\"connectorIds\":[\"In1\"]},\"type\":\"ConnectorPlacement.EquallySpacedRectSide\",\"uuid\":\"f9fadc38-a5ed-4d2c-8740-325682f7523a\"},{\"content\":{\"side\":\"RIGHT\"},\"type\":\"ConnectorPlacement.EquallySpacedRectSide\",\"uuid\":\"4cbd6435-b8f9-40e4-9703-696d88d9d9ae\"},{\"content\":{\"side\":\"TOP\"},\"type\":\"ConnectorPlacement.EquallySpacedRectSide\",\"uuid\":\"4cdd59a8-5a6d-4988-b682-29bfa74ce39c\"}]},\"type\":\"ConnectorPlacement.EquallySpacedConnector\",\"uuid\":\"f6db6523-916a-4ed8-a308-4b7cb9d0bc19\"}],\"packageUris\":[\"http://schema.mathworks.com/mf0/Connector/R2020b\"],\"version\":\"1.0\"}"
  Modularizator : Subsystem
      settings: PortSchema="{\"entries\":[{\"content\":{\"headerSize\":26,\"margin\":15,\"minimumSpacing\":25,\"sides\":[{\"content\":{\"connectorIds\":[\"In1\"]},\"type\":\"ConnectorPlacement.EquallySpacedRectSide\",\"uuid\":\"f9fadc38-a5ed-4d2c-8740-325682f7523a\"},{\"content\":{\"side\":\"RIGHT\"},\"type\":\"ConnectorPlacement.EquallySpacedRectSide\",\"uuid\":\"4cbd6435-b8f9-40e4-9703-696d88d9d9ae\"},{\"content\":{\"side\":\"TOP\"},\"type\":\"ConnectorPlacement.EquallySpacedRectSide\",\"uuid\":\"4cdd59a8-5a6d-4988-b682-29bfa74ce39c\"}]},\"type\":\"ConnectorPlacement.EquallySpacedConnector\",\"uuid\":\"f6db6523-916a-4ed8-a308-4b7cb9d0bc19\"}],\"packageUris\":[\"http://schema.mathworks.com/mf0/Connector/R2020b\"],\"version\":\"1.0\"}"
  wires:
  Bus Element In2/1 -> Modularizator/1(DisrepaireSignal)
  Bus Element In1/1 -> EnvironmentProtector/1(OceanicEnvironment)

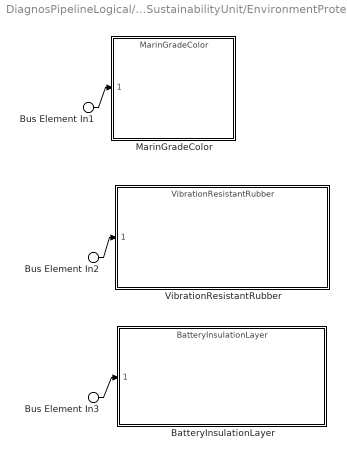
== system DiagnosPipelineLogical/SustainabilityUnit/EnvironmentProtector ==
  Bus Element In1 : Inport  PortName=OceanicEnvironment
  Bus Element In2 : Inport  PortName=OceanicEnvironment
  Bus Element In3 : Inport  PortName=OceanicEnvironment
  BatteryInsulationLayer : ModelReference  ModelNameDialog=BatteryInsulationLayer  SimulationMode=Normal  ModelReferenceVersion=1.1
      settings: PortSchema="{\"entries\":[{\"content\":{\"headerSize\":38,\"margin\":15,\"minimumSpacing\":25,\"sides\":[{\"content\":{\"connectorIds\":[\"In1\"]},\"type\":\"ConnectorPlacement.EquallySpacedRectSide\",\"uuid\":\"f9fadc38-a5ed-4d2c-8740-325682f7523a\"},{\"content\":{\"side\":\"RIGHT\"},\"type\":\"ConnectorPlacement.EquallySpacedRectSide\",\"uuid\":\"4cbd6435-b8f9-40e4-9703-696d88d9d9ae\"},{\"content\":{\"side\":\"TOP\"},\"type\":\"ConnectorPlacement.EquallySpacedRectSide\",\"uuid\":\"4cdd59a8-5a6d-4988-b682-29bfa74ce39c\"}]},\"type\":\"ConnectorPlacement.EquallySpacedConnector\",\"uuid\":\"f6db6523-916a-4ed8-a308-4b7cb9d0bc19\"}],\"packageUris\":[\"http://schema.mathworks.com/mf0/Connector/R2020b\"],\"version\":\"1.0\"}"
  MarinGradeColor : ModelReference  ModelNameDialog=MarinGradeColor  SimulationMode=Normal  ModelReferenceVersion=1.1
      settings: PortSchema="{\"entries\":[{\"content\":{\"headerSize\":38,\"margin\":15,\"minimumSpacing\":25,\"sides\":[{\"content\":{\"connectorIds\":[\"In1\"]},\"type\":\"ConnectorPlacement.EquallySpacedRectSide\",\"uuid\":\"f9fadc38-a5ed-4d2c-8740-325682f7523a\"},{\"content\":{\"side\":\"RIGHT\"},\"type\":\"ConnectorPlacement.EquallySpacedRectSide\",\"uuid\":\"4cbd6435-b8f9-40e4-9703-696d88d9d9ae\"},{\"content\":{\"side\":\"TOP\"},\"type\":\"ConnectorPlacement.EquallySpacedRectSide\",\"uuid\":\"4cdd59a8-5a6d-4988-b682-29bfa74ce39c\"}]},\"type\":\"ConnectorPlacement.EquallySpacedConnector\",\"uuid\":\"f6db6523-916a-4ed8-a308-4b7cb9d0bc19\"}],\"packageUris\":[\"http://schema.mathworks.com/mf0/Connector/R2020b\"],\"version\":\"1.0\"}"
  VibrationResistantRubber : ModelReference  ModelNameDialog=VibrationResistantRubber  SimulationMode=Normal  ModelReferenceVersion=1.1
      settings: PortSchema="{\"entries\":[{\"content\":{\"headerSize\":38,\"margin\":15,\"minimumSpacing\":25,\"sides\":[{\"content\":{\"connectorIds\":[\"In1\"]},\"type\":\"ConnectorPlacement.EquallySpacedRectSide\",\"uuid\":\"f9fadc38-a5ed-4d2c-8740-325682f7523a\"},{\"content\":{\"side\":\"RIGHT\"},\"type\":\"ConnectorPlacement.EquallySpacedRectSide\",\"uuid\":\"4cbd6435-b8f9-40e4-9703-696d88d9d9ae\"},{\"content\":{\"side\":\"TOP\"},\"type\":\"ConnectorPlacement.EquallySpacedRectSide\",\"uuid\":\"4cdd59a8-5a6d-4988-b682-29bfa74ce39c\"}]},\"type\":\"ConnectorPlacement.EquallySpacedConnector\",\"uuid\":\"f6db6523-916a-4ed8-a308-4b7cb9d0bc19\"}],\"packageUris\":[\"http://schema.mathworks.com/mf0/Connector/R2020b\"],\"version\":\"1.0\"}"
  wires:
  Bus Element In1/1 -> MarinGradeColor/1
  Bus Element In2/1 -> VibrationResistantRubber/1
  Bus Element In3/1 -> BatteryInsulationLayer/1

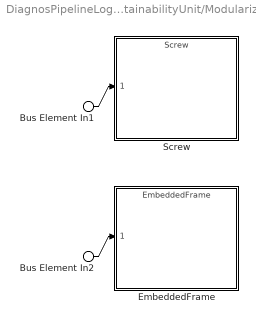
== system DiagnosPipelineLogical/SustainabilityUnit/Modularizator ==
  Bus Element In1 : Inport  PortName=DisrepaireSignal
  Bus Element In2 : Inport  PortName=DisrepaireSignal
  EmbeddedFrame : ModelReference  ModelNameDialog=EmbeddedFrame  SimulationMode=Normal  ModelReferenceVersion=1.1
      settings: PortSchema="{\"entries\":[{\"content\":{\"headerSize\":38,\"margin\":15,\"minimumSpacing\":25,\"sides\":[{\"content\":{\"connectorIds\":[\"In1\"]},\"type\":\"ConnectorPlacement.EquallySpacedRectSide\",\"uuid\":\"f9fadc38-a5ed-4d2c-8740-325682f7523a\"},{\"content\":{\"side\":\"RIGHT\"},\"type\":\"ConnectorPlacement.EquallySpacedRectSide\",\"uuid\":\"4cbd6435-b8f9-40e4-9703-696d88d9d9ae\"},{\"content\":{\"side\":\"TOP\"},\"type\":\"ConnectorPlacement.EquallySpacedRectSide\",\"uuid\":\"4cdd59a8-5a6d-4988-b682-29bfa74ce39c\"}]},\"type\":\"ConnectorPlacement.EquallySpacedConnector\",\"uuid\":\"f6db6523-916a-4ed8-a308-4b7cb9d0bc19\"}],\"packageUris\":[\"http://schema.mathworks.com/mf0/Connector/R2020b\"],\"version\":\"1.0\"}"
  Screw : ModelReference  ModelNameDialog=Screw  SimulationMode=Normal  ModelReferenceVersion=1.1
      settings: PortSchema="{\"entries\":[{\"content\":{\"headerSize\":38,\"margin\":15,\"minimumSpacing\":25,\"sides\":[{\"content\":{\"connectorIds\":[\"In1\"]},\"type\":\"ConnectorPlacement.EquallySpacedRectSide\",\"uuid\":\"f9fadc38-a5ed-4d2c-8740-325682f7523a\"},{\"content\":{\"side\":\"RIGHT\"},\"type\":\"ConnectorPlacement.EquallySpacedRectSide\",\"uuid\":\"4cbd6435-b8f9-40e4-9703-696d88d9d9ae\"},{\"content\":{\"side\":\"TOP\"},\"type\":\"ConnectorPlacement.EquallySpacedRectSide\",\"uuid\":\"4cdd59a8-5a6d-4988-b682-29bfa74ce39c\"}]},\"type\":\"ConnectorPlacement.EquallySpacedConnector\",\"uuid\":\"f6db6523-916a-4ed8-a308-4b7cb9d0bc19\"}],\"packageUris\":[\"http://schema.mathworks.com/mf0/Connector/R2020b\"],\"version\":\"1.0\"}"
  wires:
  Bus Element In1/1 -> Screw/1
  Bus Element In2/1 -> EmbeddedFrame/1
